simulink model "test_xaui_delay"  (Simulink 7.4)
settings: Solver=ode45  StartTime=0.0  StopTime=100  RelTol=1e-3
undefined symbols (not defined in the file): ROACH
libraries: xbsIndex_r4 x55, xps_library x14, casper_library x5, isi_correlator_lib x4
settings Model: Creator=wjm  LastModifiedBy=wjm
settings OptimizationCC: InitFltsAndDblsToZero=on

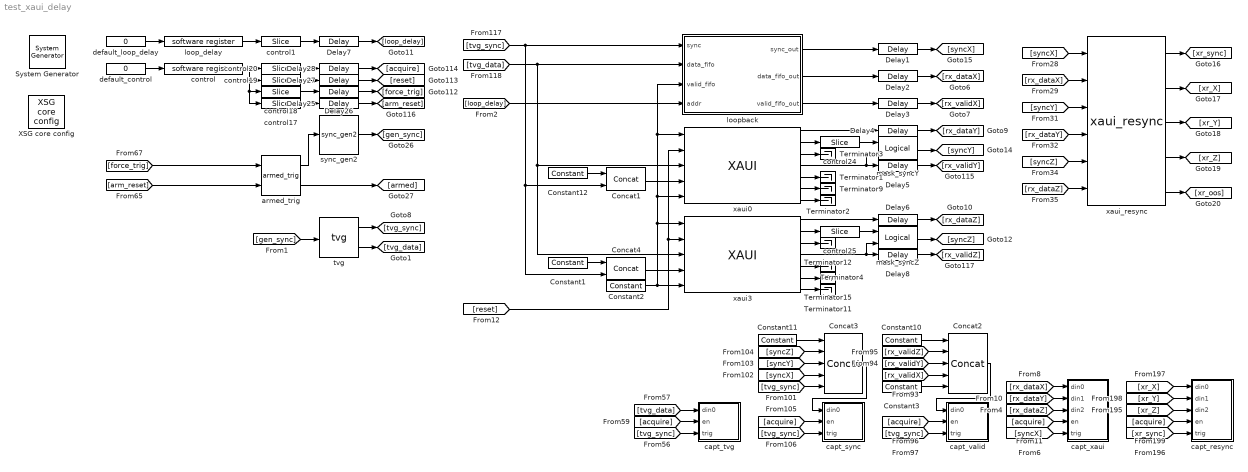
== system test_xaui_delay ==
  " System Generator" : xbsIndex_r4/ System Generator  Tag=genX  SystemSampleTime=-1  xilinxfamily=virtex5  part=xc5vsx95t  speed=-1  package=ff1136  synthesis_tool=XST  clock_wrapper=Clock Enables  directory=./test_xaui_delay/sysgen  testbench=off  simulink_period=1  sysclk_period=5  dcm_input_clock_period=100  incr_netlist=off  trim_vbits=Everywhere in SubSystem  dbl_ovrd=According to Block Masks  core_generation=According to Block Masks  run_coregen=off  deprecated_control=off  eval_field=0  block_type=sysgen
      settings: block_version=10.1.1
  Concat1 : xbsIndex_r4/Concat  num_inputs=2  dbl_ovrd=off  block_type=concat
      settings: block_version=11.3
  Concat2 : xbsIndex_r4/Concat  num_inputs=5  dbl_ovrd=off  block_type=concat
      settings: block_version=11.3
  Concat3 : xbsIndex_r4/Concat  num_inputs=5  dbl_ovrd=off  block_type=concat
      settings: block_version=11.3
  Concat4 : xbsIndex_r4/Concat  num_inputs=2  dbl_ovrd=off  block_type=concat
      settings: block_version=11.3
  Constant1 : xbsIndex_r4/Constant  arith_type=Unsigned  const=0  n_bits=3  bin_pt=0  explicit_period=on  period=1  equ=P=C  opselect=C  inp2=PCIN>>17  opr=+  inp1=P  carry=CIN  dbl_ovrd=off  block_type=constant
      settings: block_version=10.1.1
  Constant10 : xbsIndex_r4/Constant  arith_type=Unsigned  const=0  n_bits=28  bin_pt=0  explicit_period=on  period=1  equ=P=C  opselect=C  inp2=PCIN>>17  opr=+  inp1=P  carry=CIN  dbl_ovrd=off  block_type=constant
      settings: block_version=10.1.1
  Constant11 : xbsIndex_r4/Constant  arith_type=Unsigned  const=0  n_bits=28  bin_pt=0  explicit_period=on  period=1  equ=P=C  opselect=C  inp2=PCIN>>17  opr=+  inp1=P  carry=CIN  dbl_ovrd=off  block_type=constant
      settings: block_version=10.1.1
  Constant12 : xbsIndex_r4/Constant  arith_type=Unsigned  const=0  n_bits=3  bin_pt=0  explicit_period=on  period=1  equ=P=C  opselect=C  inp2=PCIN>>17  opr=+  inp1=P  carry=CIN  dbl_ovrd=off  block_type=constant
      settings: block_version=10.1.1
  Constant2 : xbsIndex_r4/Constant  arith_type=Boolean  const=1  n_bits=1  bin_pt=0  explicit_period=on  period=1  equ=P=C  opselect=C  inp2=PCIN>>17  opr=+  inp1=P  carry=CIN  dbl_ovrd=off  block_type=constant
      settings: block_version=10.1.1
  Constant3 : xbsIndex_r4/Constant  arith_type=Boolean  const=1  n_bits=1  bin_pt=0  explicit_period=on  period=1  equ=P=C  opselect=C  inp2=PCIN>>17  opr=+  inp1=P  carry=CIN  dbl_ovrd=off  block_type=constant
      settings: block_version=10.1.1
  Delay{1..8,25..28} (12 alike) : xbsIndex_r4/Delay  en=off  latency=1  dbl_ovrd=off  reg_retiming=on  block_type=delay
  Terminator{1..4,9,11..12,15} (8 alike) : Terminator
  XSG core config : xps_library/XSG core config  Tag=xps:xsg  SystemSampleTime=-1  hw_sys=ROACH:sx95t  ibob_linux=off  clk_src=sys_clk2x  iBOB_clk_src=sys_clk  BEE2_ctrl_clk_src=sys_clk  BEE2_usr_clk_src=sys_clk  ROACH_clk_src=sys_clk2x  CORR_clk_src=sys_clk  gpio_clk_io_group=iBOB:sma  gpio_clk_bit_index=0  clk_rate=200  sample_period=1  synthesis_tool=XST  mpc_type=powerpc440_ext
  armed_trig : isi_correlator_lib/armed_trig  SystemSampleTime=-1
  capt_resync : Subsystem  AncestorBlock=isi_correlator_lib/capture  mask(capture){num_brams=3, addr_width=11, done_port=off}
      mask prompts: num_brams "Number of BRAMs:"; addr_width "Address width:"; done_port "Provide done port"
      mask help: This block captures N data lines into N separate BRAMs.
      mask init:
      | capture_init(gcb, ...
      |     'num_brams', num_brams, ...
      |     'addr_width', addr_width, ...
      |     'done_port', done_port);
  capt_sync : Subsystem  AncestorBlock=isi_correlator_lib/capture  mask(capture){num_brams=1, addr_width=11, done_port=off}
      mask prompts: num_brams "Number of BRAMs:"; addr_width "Address width:"; done_port "Provide done port"
      mask help: This block captures N data lines into N separate BRAMs.
      mask init:
      | capture_init(gcb, ...
      |     'num_brams', num_brams, ...
      |     'addr_width', addr_width, ...
      |     'done_port', done_port);
  capt_tvg : Subsystem  AncestorBlock=isi_correlator_lib/capture  mask(capture){num_brams=1, addr_width=11, done_port=off}
      mask prompts: num_brams "Number of BRAMs:"; addr_width "Address width:"; done_port "Provide done port"
      mask help: This block captures N data lines into N separate BRAMs.
      mask init:
      | capture_init(gcb, ...
      |     'num_brams', num_brams, ...
      |     'addr_width', addr_width, ...
      |     'done_port', done_port);
  capt_valid : Subsystem  AncestorBlock=isi_correlator_lib/capture  mask(capture){num_brams=1, addr_width=11, done_port=off}
      mask prompts: num_brams "Number of BRAMs:"; addr_width "Address width:"; done_port "Provide done port"
      mask help: This block captures N data lines into N separate BRAMs.
      mask init:
      | capture_init(gcb, ...
      |     'num_brams', num_brams, ...
      |     'addr_width', addr_width, ...
      |     'done_port', done_port);
  capt_xaui : Subsystem  AncestorBlock=isi_correlator_lib/capture  mask(capture){num_brams=3, addr_width=11, done_port=off}
      mask prompts: num_brams "Number of BRAMs:"; addr_width "Address width:"; done_port "Provide done port"
      mask help: This block captures N data lines into N separate BRAMs.
      mask init:
      | capture_init(gcb, ...
      |     'num_brams', num_brams, ...
      |     'addr_width', addr_width, ...
      |     'done_port', done_port);
  control : xps_library/software register  Tag=xps:sw_reg  SystemSampleTime=-1  io_dir=From Processor  arith_type=Unsigned  bitwidth=32  bin_pt=0  sample_period=1  gw_name=test_xaui_delay_control_user_data_out
  control1 : xbsIndex_r4/Slice  nbits=10  boolean_output=off  mode=Lower Bit Location + Width  bit1=0  base1=MSB of Input  bit0=0  base0=LSB of Input  dbl_ovrd=off  block_type=slice
      settings: block_version=10.1.3
  control17 : xbsIndex_r4/Slice  nbits=1  boolean_output=on  mode=Lower Bit Location + Width  bit1=0  base1=MSB of Input  bit0=0  base0=LSB of Input  dbl_ovrd=off  block_type=slice
      settings: infoedit="Extracts a given range of bits from each input sample and presents it at the output.  The output type is ordinarily unsigned with binary point at zero, but can be Boolean when the slice is one bit wide.<P><P>Hardware notes: In hardware this block costs nothing."  block_version=10.1.3
  control18 : xbsIndex_r4/Slice  nbits=1  boolean_output=on  mode=Lower Bit Location + Width  bit1=0  base1=MSB of Input  bit0=1  base0=LSB of Input  dbl_ovrd=off  block_type=slice
      settings: infoedit="Extracts a given range of bits from each input sample and presents it at the output.  The output type is ordinarily unsigned with binary point at zero, but can be Boolean when the slice is one bit wide.<P><P>Hardware notes: In hardware this block costs nothing."  block_version=10.1.3
  control19 : xbsIndex_r4/Slice  nbits=1  boolean_output=on  mode=Lower Bit Location + Width  bit1=0  base1=MSB of Input  bit0=2  base0=LSB of Input  dbl_ovrd=off  block_type=slice
      settings: infoedit="Extracts a given range of bits from each input sample and presents it at the output.  The output type is ordinarily unsigned with binary point at zero, but can be Boolean when the slice is one bit wide.<P><P>Hardware notes: In hardware this block costs nothing."  block_version=10.1.3
  control20 : xbsIndex_r4/Slice  nbits=1  boolean_output=on  mode=Lower Bit Location + Width  bit1=0  base1=MSB of Input  bit0=3  base0=LSB of Input  dbl_ovrd=off  block_type=slice
      settings: infoedit="Extracts a given range of bits from each input sample and presents it at the output.  The output type is ordinarily unsigned with binary point at zero, but can be Boolean when the slice is one bit wide.<P><P>Hardware notes: In hardware this block costs nothing."  block_version=10.1.3
  control24 : xbsIndex_r4/Slice  nbits=1  boolean_output=on  mode=Lower Bit Location + Width  bit1=0  base1=MSB of Input  bit0=0  base0=LSB of Input  dbl_ovrd=off  block_type=slice
      settings: infoedit="Extracts a given range of bits from each input sample and presents it at the output.  The output type is ordinarily unsigned with binary point at zero, but can be Boolean when the slice is one bit wide.<P><P>Hardware notes: In hardware this block costs nothing."  block_version=10.1.3
  control25 : xbsIndex_r4/Slice  nbits=1  boolean_output=on  mode=Lower Bit Location + Width  bit1=0  base1=MSB of Input  bit0=0  base0=LSB of Input  dbl_ovrd=off  block_type=slice
      settings: infoedit="Extracts a given range of bits from each input sample and presents it at the output.  The output type is ordinarily unsigned with binary point at zero, but can be Boolean when the slice is one bit wide.<P><P>Hardware notes: In hardware this block costs nothing."  block_version=10.1.3
  default_control : Constant  Value=0  OutDataType=sfix(16)  OutScaling=2^0  SampleTime=1
  default_loop_delay : Constant  Value=0  OutDataType=sfix(16)  OutScaling=2^0  SampleTime=1
  loop_delay : xps_library/software register  Tag=xps:sw_reg  SystemSampleTime=-1  io_dir=From Processor  arith_type=Unsigned  bitwidth=32  bin_pt=0  sample_period=1  gw_name=test_xaui_delay_loop_delay_user_data_out
  loopback : Subsystem
  mask_syncY : xbsIndex_r4/Logical  logical_function=AND  inputs=2  en=off  latency=1  precision=Full  arith_type=Unsigned  n_bits=16  bin_pt=0  align_bp=on  dbl_ovrd=off  block_type=logical
      settings: block_version=11.4
  mask_syncZ : xbsIndex_r4/Logical  logical_function=AND  inputs=2  en=off  latency=1  precision=Full  arith_type=Unsigned  n_bits=16  bin_pt=0  align_bp=on  dbl_ovrd=off  block_type=logical
      settings: block_version=11.4
  sync_gen2 : isi_correlator_lib/sync_gen2  SystemSampleTime=-1
  tvg : isi_correlator_lib/tvg  SystemSampleTime=-1  addr_width=11
  xaui0 : xps_library/XAUI  Tag=xps:xaui  SystemSampleTime=-1  demux=2  port=ROACH:0  open_phy=on  show_param=off  pre_emph=3  swing=800
  xaui3 : xps_library/XAUI  Tag=xps:xaui  SystemSampleTime=-1  demux=2  port=ROACH:3  open_phy=on  show_param=off  pre_emph=3  swing=800
  xaui_resync : isi_correlator_lib/xaui_resync  SystemSampleTime=-1  buffer_depth=10  logic_latency=1
  wires:
  [xr_Y] -> capt_resync/2(din1)
  [xr_Z] -> capt_resync/3(din2)
  [acquire] -> capt_resync/4(en)
  [xr_sync] -> capt_resync/5(trig)
  [arm_reset] -> armed_trig/2
  [force_trig] -> armed_trig/1
  armed_trig/1 -> sync_gen2/1
  armed_trig/2 -> [armed]
  sync_gen2/1 -> [gen_sync]
  control20/1 -> Delay28/1
  control19/1 -> Delay27/1
  control18/1 -> Delay26/1
  control17/1 -> Delay25/1
  Delay26/1 -> [force_trig]
  Delay27/1 -> [reset]
  Delay28/1 -> [acquire]
  default_control/1 -> control/1
  Delay25/1 -> [arm_reset]
  [rx_dataY] -> capt_xaui/2(din1)
  [rx_dataZ] -> capt_xaui/3(din2)
  [acquire] -> capt_xaui/4(en)
  [syncX] -> capt_xaui/5(trig)
  [rx_dataX] -> capt_xaui/1(din0)
  Concat2/1 -> capt_valid/1(din0)
  [acquire] -> capt_valid/2(en)
  [tvg_sync] -> capt_valid/3(trig)
  Constant10/1 -> Concat2/1
  [rx_validZ] -> Concat2/2
  [rx_validY] -> Concat2/3
  [rx_validX] -> Concat2/4
  Constant3/1 -> Concat2/5
  Concat3/1 -> capt_sync/1(din0)
  [xr_X] -> capt_resync/1(din0)
  control/1 -> control20/1, control19/1, control17/1, control18/1
  [gen_sync] -> tvg/1
  tvg/2 -> [tvg_data]
  tvg/1 -> [tvg_sync]
  Constant11/1 -> Concat3/1
  [syncX] -> Concat3/4
  [tvg_sync] -> Concat3/5
  [acquire] -> capt_sync/2(en)
  [syncY] -> Concat3/3
  [syncZ] -> Concat3/2
  default_loop_delay/1 -> loop_delay/1
  loop_delay/1 -> control1/1
  Delay7/1 -> [loop_delay]
  [tvg_sync] -> loopback/1(sync), Concat4/2, Concat1/2
  [tvg_data] -> loopback/2(data_fifo), xaui3/3, xaui0/3
  xaui0/1 -> Delay4/1
  xaui0/3 -> Terminator3/1
  xaui0/4 -> mask_syncY/2, Delay5/1
  xaui0/5 -> Terminator1/1
  xaui0/6 -> Terminator9/1
  xaui0/7 -> Terminator2/1
  xaui3/1 -> Delay6/1
  xaui3/2 -> control25/1
  xaui3/3 -> Terminator12/1
  xaui3/4 -> mask_syncZ/2, Delay8/1
  xaui3/5 -> Terminator4/1
  xaui3/6 -> Terminator15/1
  xaui3/7 -> Terminator11/1
  loopback/2(data_fifo_out) -> Delay2/1
  loopback/3(valid_fifo_out) -> Delay3/1
  loopback/1(sync_out) -> Delay1/1
  mask_syncZ/1 -> [syncZ]
  mask_syncY/1 -> [syncY]
  control25/1 -> mask_syncZ/1
  xaui0/2 -> control24/1
  control24/1 -> mask_syncY/1
  Constant1/1 -> Concat4/1
  Concat4/1 -> xaui3/4
  [reset] -> xaui0/2, xaui3/2
  Constant12/1 -> Concat1/1
  Concat1/1 -> xaui0/4
  [syncX] -> xaui_resync/1
  [rx_dataX] -> xaui_resync/2
  [syncY] -> xaui_resync/3
  [rx_dataY] -> xaui_resync/4
  [syncZ] -> xaui_resync/5
  [rx_dataZ] -> xaui_resync/6
  xaui_resync/1 -> [xr_sync]
  xaui_resync/2 -> [xr_X]
  xaui_resync/3 -> [xr_Y]
  xaui_resync/4 -> [xr_Z]
  xaui_resync/5 -> [xr_oos]
  [acquire] -> capt_tvg/2(en)
  [tvg_sync] -> capt_tvg/3(trig)
  Constant2/1 -> xaui3/5, xaui3/1, loopback/3(valid_fifo), xaui0/1, xaui0/5
  [loop_delay] -> loopback/4(addr)
  control1/1 -> Delay7/1
  [tvg_sync] -> capt_sync/3(trig)
  [tvg_data] -> capt_tvg/1(din0)
  Delay1/1 -> [syncX]
  Delay2/1 -> [rx_dataX]
  Delay3/1 -> [rx_validX]
  Delay4/1 -> [rx_dataY]
  Delay5/1 -> [rx_validY]
  Delay6/1 -> [rx_dataZ]
  Delay8/1 -> [rx_validZ]

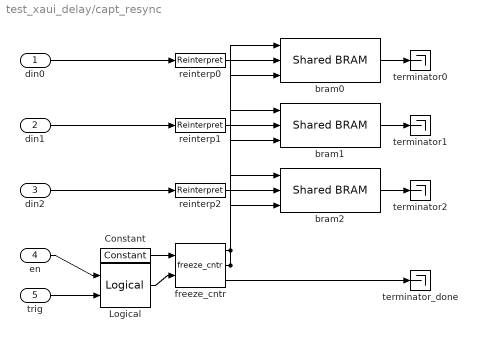
== system test_xaui_delay/capt_resync ==
  din0 : Inport
  din1 : Inport  Port=2
  din2 : Inport  Port=3
  en : Inport  Port=4
  trig : Inport  Port=5
  Constant : xbsIndex_r4/Constant  arith_type=Boolean  const=1  n_bits=1  bin_pt=0  explicit_period=on  period=1  equ=P=C  opselect=C  inp2=PCIN>>17  opr=+  inp1=P  carry=CIN  dbl_ovrd=off  block_type=constant
      settings: block_version=11.3
  Logical : xbsIndex_r4/Logical  logical_function=AND  inputs=2  en=off  latency=0  precision=Full  arith_type=Unsigned  n_bits=16  bin_pt=0  align_bp=on  dbl_ovrd=off  block_type=logical
      settings: block_version=11.3
  bram0 : xps_library/Shared BRAM  Tag=xps:bram  SystemSampleTime=-1  arith_type=Unsigned  addr_width=addr_width  data_width=32  data_bin_pt=0  init_vals=0  sample_rate=1
  bram1 : xps_library/Shared BRAM  Tag=xps:bram  SystemSampleTime=-1  arith_type=Unsigned  addr_width=addr_width  data_width=32  data_bin_pt=0  init_vals=0  sample_rate=1
  bram2 : xps_library/Shared BRAM  Tag=xps:bram  SystemSampleTime=-1  arith_type=Unsigned  addr_width=addr_width  data_width=32  data_bin_pt=0  init_vals=0  sample_rate=1
  freeze_cntr : casper_library/Misc/freeze_cntr  SystemSampleTime=-1  CounterBits=addr_width
  reinterp0 : xbsIndex_r4/Reinterpret  force_arith_type=on  arith_type=Unsigned  force_bin_pt=on  bin_pt=0  block_type=reinterpret
      settings: infoedit="Changes signal type without altering the binary representation.   You can changed the signal between signed and unsigned, and relocate the binary point.<br><br>Hardware notes: In hardware this block costs nothing.<br><br>Example:  Suppose the input is 6 bits wide, signed, with 2 fractional bits, and the output is forced to unsigned with 0 fractional bits.  Then an input of -2.0 (1110.00 in binary 2's complement) becomes an output of 56 (111000 in binary)."  block_version=11.3
  reinterp1 : xbsIndex_r4/Reinterpret  force_arith_type=on  arith_type=Unsigned  force_bin_pt=on  bin_pt=0  block_type=reinterpret
      settings: infoedit="Changes signal type without altering the binary representation.   You can changed the signal between signed and unsigned, and relocate the binary point.<br><br>Hardware notes: In hardware this block costs nothing.<br><br>Example:  Suppose the input is 6 bits wide, signed, with 2 fractional bits, and the output is forced to unsigned with 0 fractional bits.  Then an input of -2.0 (1110.00 in binary 2's complement) becomes an output of 56 (111000 in binary)."  block_version=11.3
  reinterp2 : xbsIndex_r4/Reinterpret  force_arith_type=on  arith_type=Unsigned  force_bin_pt=on  bin_pt=0  block_type=reinterpret
      settings: infoedit="Changes signal type without altering the binary representation.   You can changed the signal between signed and unsigned, and relocate the binary point.<br><br>Hardware notes: In hardware this block costs nothing.<br><br>Example:  Suppose the input is 6 bits wide, signed, with 2 fractional bits, and the output is forced to unsigned with 0 fractional bits.  Then an input of -2.0 (1110.00 in binary 2's complement) becomes an output of 56 (111000 in binary)."  block_version=11.3
  terminator0 : Terminator
  terminator1 : Terminator
  terminator2 : Terminator
  terminator_done : Terminator
  wires:
  freeze_cntr/2 -> bram2/3, bram1/3, bram0/3
  freeze_cntr/1 -> bram2/1, bram1/1, bram0/1
  Logical/1 -> freeze_cntr/2
  Constant/1 -> freeze_cntr/1
  trig/1 -> Logical/2
  en/1 -> Logical/1
  freeze_cntr/3 -> terminator_done/1
  bram2/1 -> terminator2/1
  reinterp2/1 -> bram2/2
  din2/1 -> reinterp2/1
  bram1/1 -> terminator1/1
  reinterp1/1 -> bram1/2
  din1/1 -> reinterp1/1
  bram0/1 -> terminator0/1
  reinterp0/1 -> bram0/2
  din0/1 -> reinterp0/1

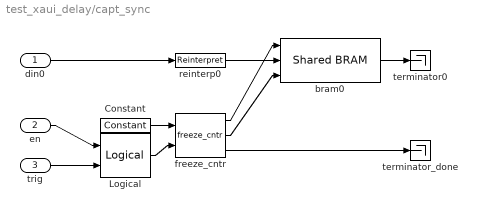
== system test_xaui_delay/capt_sync ==
  din0 : Inport
  en : Inport  Port=2
  trig : Inport  Port=3
  Constant : xbsIndex_r4/Constant  arith_type=Boolean  const=1  n_bits=1  bin_pt=0  explicit_period=on  period=1  equ=P=C  opselect=C  inp2=PCIN>>17  opr=+  inp1=P  carry=CIN  dbl_ovrd=off  block_type=constant
      settings: block_version=11.3
  Logical : xbsIndex_r4/Logical  logical_function=AND  inputs=2  en=off  latency=0  precision=Full  arith_type=Unsigned  n_bits=16  bin_pt=0  align_bp=on  dbl_ovrd=off  block_type=logical
      settings: block_version=11.3
  bram0 : xps_library/Shared BRAM  Tag=xps:bram  SystemSampleTime=-1  arith_type=Unsigned  addr_width=addr_width  data_width=32  data_bin_pt=0  init_vals=0  sample_rate=1
  freeze_cntr : casper_library/Misc/freeze_cntr  SystemSampleTime=-1  CounterBits=addr_width
  reinterp0 : xbsIndex_r4/Reinterpret  force_arith_type=on  arith_type=Unsigned  force_bin_pt=on  bin_pt=0  block_type=reinterpret
      settings: infoedit="Changes signal type without altering the binary representation.   You can changed the signal between signed and unsigned, and relocate the binary point.<br><br>Hardware notes: In hardware this block costs nothing.<br><br>Example:  Suppose the input is 6 bits wide, signed, with 2 fractional bits, and the output is forced to unsigned with 0 fractional bits.  Then an input of -2.0 (1110.00 in binary 2's complement) becomes an output of 56 (111000 in binary)."  block_version=11.3
  terminator0 : Terminator
  terminator_done : Terminator
  wires:
  freeze_cntr/2 -> bram0/3
  freeze_cntr/1 -> bram0/1
  Logical/1 -> freeze_cntr/2
  Constant/1 -> freeze_cntr/1
  trig/1 -> Logical/2
  en/1 -> Logical/1
  freeze_cntr/3 -> terminator_done/1
  bram0/1 -> terminator0/1
  reinterp0/1 -> bram0/2
  din0/1 -> reinterp0/1

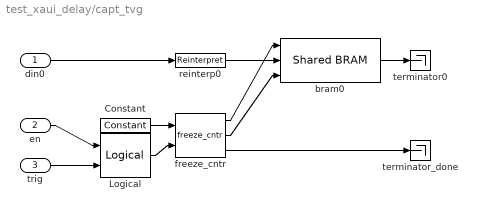
== system test_xaui_delay/capt_tvg ==
  din0 : Inport
  en : Inport  Port=2
  trig : Inport  Port=3
  Constant : xbsIndex_r4/Constant  arith_type=Boolean  const=1  n_bits=1  bin_pt=0  explicit_period=on  period=1  equ=P=C  opselect=C  inp2=PCIN>>17  opr=+  inp1=P  carry=CIN  dbl_ovrd=off  block_type=constant
      settings: block_version=11.3
  Logical : xbsIndex_r4/Logical  logical_function=AND  inputs=2  en=off  latency=0  precision=Full  arith_type=Unsigned  n_bits=16  bin_pt=0  align_bp=on  dbl_ovrd=off  block_type=logical
      settings: block_version=11.3
  bram0 : xps_library/Shared BRAM  Tag=xps:bram  SystemSampleTime=-1  arith_type=Unsigned  addr_width=addr_width  data_width=32  data_bin_pt=0  init_vals=0  sample_rate=1
  freeze_cntr : casper_library/Misc/freeze_cntr  SystemSampleTime=-1  CounterBits=addr_width
  reinterp0 : xbsIndex_r4/Reinterpret  force_arith_type=on  arith_type=Unsigned  force_bin_pt=on  bin_pt=0  block_type=reinterpret
      settings: infoedit="Changes signal type without altering the binary representation.   You can changed the signal between signed and unsigned, and relocate the binary point.<br><br>Hardware notes: In hardware this block costs nothing.<br><br>Example:  Suppose the input is 6 bits wide, signed, with 2 fractional bits, and the output is forced to unsigned with 0 fractional bits.  Then an input of -2.0 (1110.00 in binary 2's complement) becomes an output of 56 (111000 in binary)."  block_version=11.3
  terminator0 : Terminator
  terminator_done : Terminator
  wires:
  freeze_cntr/2 -> bram0/3
  freeze_cntr/1 -> bram0/1
  Logical/1 -> freeze_cntr/2
  Constant/1 -> freeze_cntr/1
  trig/1 -> Logical/2
  en/1 -> Logical/1
  freeze_cntr/3 -> terminator_done/1
  bram0/1 -> terminator0/1
  reinterp0/1 -> bram0/2
  din0/1 -> reinterp0/1

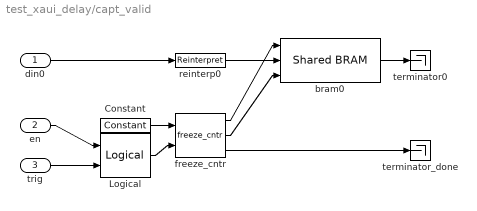
== system test_xaui_delay/capt_valid ==
  din0 : Inport
  en : Inport  Port=2
  trig : Inport  Port=3
  Constant : xbsIndex_r4/Constant  arith_type=Boolean  const=1  n_bits=1  bin_pt=0  explicit_period=on  period=1  equ=P=C  opselect=C  inp2=PCIN>>17  opr=+  inp1=P  carry=CIN  dbl_ovrd=off  block_type=constant
      settings: block_version=11.3
  Logical : xbsIndex_r4/Logical  logical_function=AND  inputs=2  en=off  latency=0  precision=Full  arith_type=Unsigned  n_bits=16  bin_pt=0  align_bp=on  dbl_ovrd=off  block_type=logical
      settings: block_version=11.3
  bram0 : xps_library/Shared BRAM  Tag=xps:bram  SystemSampleTime=-1  arith_type=Unsigned  addr_width=addr_width  data_width=32  data_bin_pt=0  init_vals=0  sample_rate=1
  freeze_cntr : casper_library/Misc/freeze_cntr  SystemSampleTime=-1  CounterBits=addr_width
  reinterp0 : xbsIndex_r4/Reinterpret  force_arith_type=on  arith_type=Unsigned  force_bin_pt=on  bin_pt=0  block_type=reinterpret
      settings: infoedit="Changes signal type without altering the binary representation.   You can changed the signal between signed and unsigned, and relocate the binary point.<br><br>Hardware notes: In hardware this block costs nothing.<br><br>Example:  Suppose the input is 6 bits wide, signed, with 2 fractional bits, and the output is forced to unsigned with 0 fractional bits.  Then an input of -2.0 (1110.00 in binary 2's complement) becomes an output of 56 (111000 in binary)."  block_version=11.3
  terminator0 : Terminator
  terminator_done : Terminator
  wires:
  din0/1 -> reinterp0/1
  reinterp0/1 -> bram0/2
  bram0/1 -> terminator0/1
  freeze_cntr/3 -> terminator_done/1
  en/1 -> Logical/1
  trig/1 -> Logical/2
  Constant/1 -> freeze_cntr/1
  Logical/1 -> freeze_cntr/2
  freeze_cntr/1 -> bram0/1
  freeze_cntr/2 -> bram0/3

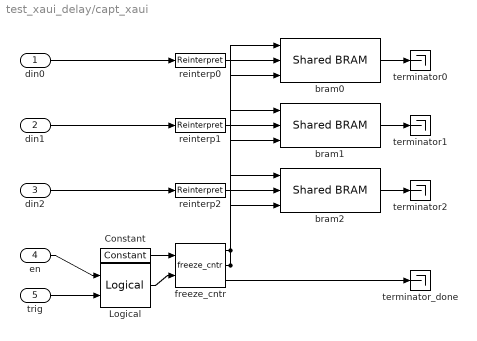
== system test_xaui_delay/capt_xaui ==
  din0 : Inport
  din1 : Inport  Port=2
  din2 : Inport  Port=3
  en : Inport  Port=4
  trig : Inport  Port=5
  Constant : xbsIndex_r4/Constant  arith_type=Boolean  const=1  n_bits=1  bin_pt=0  explicit_period=on  period=1  equ=P=C  opselect=C  inp2=PCIN>>17  opr=+  inp1=P  carry=CIN  dbl_ovrd=off  block_type=constant
      settings: block_version=11.3
  Logical : xbsIndex_r4/Logical  logical_function=AND  inputs=2  en=off  latency=0  precision=Full  arith_type=Unsigned  n_bits=16  bin_pt=0  align_bp=on  dbl_ovrd=off  block_type=logical
      settings: block_version=11.3
  bram0 : xps_library/Shared BRAM  Tag=xps:bram  SystemSampleTime=-1  arith_type=Unsigned  addr_width=addr_width  data_width=32  data_bin_pt=0  init_vals=0  sample_rate=1
  bram1 : xps_library/Shared BRAM  Tag=xps:bram  SystemSampleTime=-1  arith_type=Unsigned  addr_width=addr_width  data_width=32  data_bin_pt=0  init_vals=0  sample_rate=1
  bram2 : xps_library/Shared BRAM  Tag=xps:bram  SystemSampleTime=-1  arith_type=Unsigned  addr_width=addr_width  data_width=32  data_bin_pt=0  init_vals=0  sample_rate=1
  freeze_cntr : casper_library/Misc/freeze_cntr  SystemSampleTime=-1  CounterBits=addr_width
  reinterp0 : xbsIndex_r4/Reinterpret  force_arith_type=on  arith_type=Unsigned  force_bin_pt=on  bin_pt=0  block_type=reinterpret
      settings: infoedit="Changes signal type without altering the binary representation.   You can changed the signal between signed and unsigned, and relocate the binary point.<br><br>Hardware notes: In hardware this block costs nothing.<br><br>Example:  Suppose the input is 6 bits wide, signed, with 2 fractional bits, and the output is forced to unsigned with 0 fractional bits.  Then an input of -2.0 (1110.00 in binary 2's complement) becomes an output of 56 (111000 in binary)."  block_version=11.3
  reinterp1 : xbsIndex_r4/Reinterpret  force_arith_type=on  arith_type=Unsigned  force_bin_pt=on  bin_pt=0  block_type=reinterpret
      settings: infoedit="Changes signal type without altering the binary representation.   You can changed the signal between signed and unsigned, and relocate the binary point.<br><br>Hardware notes: In hardware this block costs nothing.<br><br>Example:  Suppose the input is 6 bits wide, signed, with 2 fractional bits, and the output is forced to unsigned with 0 fractional bits.  Then an input of -2.0 (1110.00 in binary 2's complement) becomes an output of 56 (111000 in binary)."  block_version=11.3
  reinterp2 : xbsIndex_r4/Reinterpret  force_arith_type=on  arith_type=Unsigned  force_bin_pt=on  bin_pt=0  block_type=reinterpret
      settings: infoedit="Changes signal type without altering the binary representation.   You can changed the signal between signed and unsigned, and relocate the binary point.<br><br>Hardware notes: In hardware this block costs nothing.<br><br>Example:  Suppose the input is 6 bits wide, signed, with 2 fractional bits, and the output is forced to unsigned with 0 fractional bits.  Then an input of -2.0 (1110.00 in binary 2's complement) becomes an output of 56 (111000 in binary)."  block_version=11.3
  terminator0 : Terminator
  terminator1 : Terminator
  terminator2 : Terminator
  terminator_done : Terminator
  wires:
  din0/1 -> reinterp0/1
  reinterp0/1 -> bram0/2
  bram0/1 -> terminator0/1
  din1/1 -> reinterp1/1
  reinterp1/1 -> bram1/2
  bram1/1 -> terminator1/1
  din2/1 -> reinterp2/1
  reinterp2/1 -> bram2/2
  bram2/1 -> terminator2/1
  freeze_cntr/3 -> terminator_done/1
  en/1 -> Logical/1
  trig/1 -> Logical/2
  Constant/1 -> freeze_cntr/1
  Logical/1 -> freeze_cntr/2
  freeze_cntr/1 -> bram0/1, bram1/1, bram2/1
  freeze_cntr/2 -> bram0/3, bram1/3, bram2/3

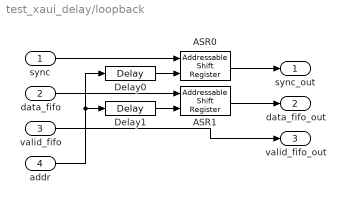
== system test_xaui_delay/loopback ==
  sync : Inport  OutDataType=sfix(16)  OutScaling=2^0
  data_fifo : Inport  Port=2  OutDataType=sfix(16)  OutScaling=2^0
  valid_fifo : Inport  Port=3  OutDataType=sfix(16)  OutScaling=2^0
  addr : Inport  Port=4  OutDataType=sfix(16)  OutScaling=2^0
  ASR0 : xbsIndex_r4/Addressable Shift Register  infer_latency=on  depth=0  initVector=[0]  en=off  dbl_ovrd=off  use_behavioral_HDL=off  block_type=addrsr
      settings: infoedit="Delay of configurable length.  Any element in the delay line can be addressed and driven onto the output port.<br><br>Hardware notes: This block is implemented using SRL16s. If Virtex-4 or Spartan-3 device is used, multiple SRLC16s are cascaded together."  block_version=11.4
  ASR1 : xbsIndex_r4/Addressable Shift Register  infer_latency=on  depth=0  initVector=[0]  en=off  dbl_ovrd=off  use_behavioral_HDL=off  block_type=addrsr
      settings: infoedit="Delay of configurable length.  Any element in the delay line can be addressed and driven onto the output port.<br><br>Hardware notes: This block is implemented using SRL16s. If Virtex-4 or Spartan-3 device is used, multiple SRLC16s are cascaded together."  block_version=11.4
  Delay0 : xbsIndex_r4/Delay  en=off  latency=2  dbl_ovrd=off  reg_retiming=on  block_type=delay
  Delay1 : xbsIndex_r4/Delay  en=off  latency=2  dbl_ovrd=off  reg_retiming=on  block_type=delay
  sync_out : Outport  OutDataType=sfix(16)  OutScaling=2^0
  data_fifo_out : Outport  Port=2  OutDataType=sfix(16)  OutScaling=2^0
  valid_fifo_out : Outport  Port=3  OutDataType=sfix(16)  OutScaling=2^0
  wires:
  sync/1 -> ASR0/1
  data_fifo/1 -> ASR1/1
  ASR0/1 -> sync_out/1
  ASR1/1 -> data_fifo_out/1
  valid_fifo/1 -> valid_fifo_out/1
  addr/1 -> Delay0/1, Delay1/1
  Delay0/1 -> ASR0/2
  Delay1/1 -> ASR1/2
